simulink model "cable_robot_2t_4cables_2019b"  (R2019b)
settings: Solver=ode3  StartTime=0.0  StopTime=tend_sim  FixedStep=stepsize  MaxStep=1e-3  RelTol=1e-3
InitFcn:
  | close all
  | clear
  | Simulink.sdi.clear
  | run scripts\init_model.m
undefined symbols (not defined in the file): DirectionOfGravity, Dy0, f_max, f_min, g, K_fc, PlatformWeight, sigbuilder_block, T_fc, tend_sim, y0
settings Model: Creator=ac123748  LastModifiedBy=rausc
settings DataIOCC: SaveOutput=off  ReturnWorkspaceOutputs=off  SignalLoggingName=tmp_raccel_logsout
settings OptimizationCC: EfficientMapNaN2IntZero=off
settings DebuggingCC: ArithmeticOperatorsInVariantConditions=warning
settings HardwareCC: TargetBitPerPointer=64  TargetBitPerSizeT=64  TargetBitPerPtrDiffT=64  TargetLongLongMode=on  TargetIntDivRoundTo=Zero  TargetEndianess=LittleEndian  TargetWordSize=64  TargetHWDeviceType=MATLAB Host  ProdEqTarget=off
settings SFSimCC: SimUseLocalCustomCode=off  CustomCodeUndefinedFunction=UseInterfaceOnly
settings RTWCC: SystemTargetFile=raccel.tlc  TemplateMakefile=raccel_default_tmf  RTWVerbose=off  RTWUseLocalCustomCode=off  RTWUseSimCustomCode=on
settings CodeAppCC: GenerateComments=off  MaxIdLength=128  SimulinkBlockComments=off
settings RaccelTargetCC: LogVarNameModifier=rt_  MultiInstanceERTCode=off  ENABLE_SLEXEC_SSBRIDGE=0  RTWCAPISignals=off  RTWCAPIParams=off  RTWCAPIRootIO=off

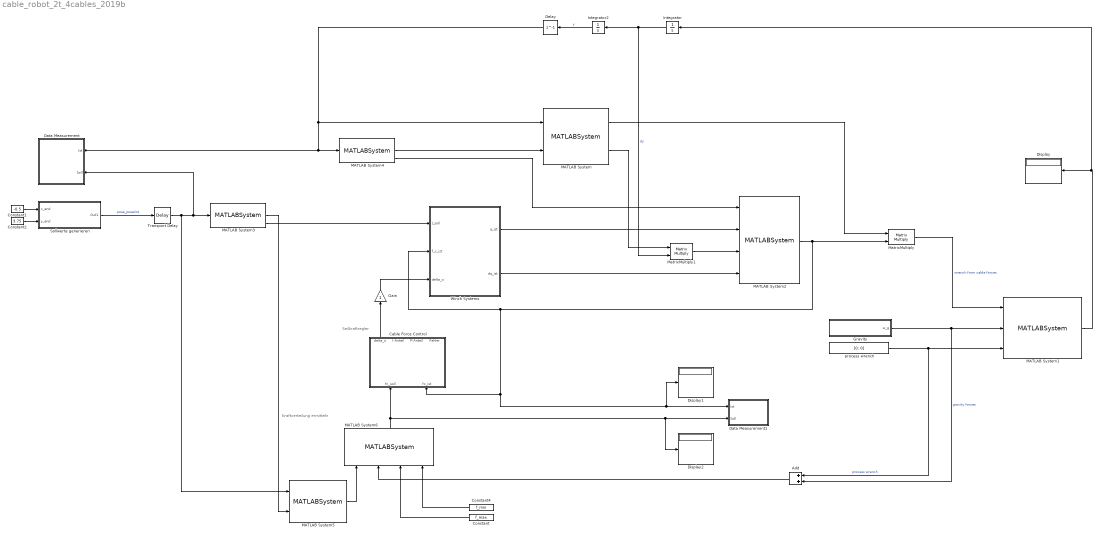
== system cable_robot_2t_4cables_2019b ==
  note: Seilkraftregler
  note: Kraftverteilung ermitteln
  Add : Sum
  Cable Force Control : Subsystem
  Constant : Constant  Value=f_max
  Constant1 : Constant  Value=-0.5
  Constant2 : Constant  Value=3.75
  Constant4 : Constant  Value=f_min
  Data Measurement : Subsystem
  Data Measurement1 : Subsystem
  Delay : Delay  DelayLength=1
  Display : Display
  Display1 : Display
  Display2 : Display
  Gain : Gain
  Gravity : Subsystem
  Integrator : Integrator  InitialCondition=Dy0
  Integrator2 : Integrator  InitialCondition=y0
  MATLAB System : MATLABSystem  System=sm.structurematrix_4cables  inv_Jacobian=on  Platform=zeros( 4, 2 )
      mask Type: sm.structurematrix_4cables
      mask Display:
      | disp('sm.structurematrix_4cables');
      | port_label('input',1,'p');
      | port_label('input',2,'u');
      | port_label('output',1,'AT');
      | port_label('output',2,'J_inv');
  MATLAB System1 : MATLABSystem  System=dynamics.platform_4cables  Weight=5
      mask Type: dynamics.platform_4cables
      mask Display:
      | disp('dynamics.platform_4cables');
      | port_label('input',1,'w_c');
      | port_label('input',2,'w_g');
      | port_label('input',3,'w_p');
      | port_label('output',1,'ddy');
  MATLAB System2 : MATLABSystem  System=cable.linearelasticity_4cables  Elasticity=172e3 * ones( 4, 1 )  Viscosity=0.03 * 172e3 * ones( 4, 1 )  Reference_Length=ones( 4, 1 )  Initial_Length=zeros( 4, 1 )  SimulateUsing=Code generation
      mask Type: cable.linearelasticity_4cables
      mask Display:
      | disp('cable.linearelasticity_4cables');
      | port_label('input',1,'l');
      | port_label('input',2,'q');
      | port_label('input',3,'dl');
      | port_label('input',4,'dq');
      | port_label('output',1,'f_c');
  MATLAB System3 : MATLABSystem  System=ik.ik_standard_4cables  UnitVectors=on  DeltaLength=on  FrameAnchors=[ [ -4.70, 4.30 ]; [ 3.70, 3.20 ]; [ 3.50, -5.20 ]; [ -4.50, -5.00 ] ]  Platform=zeros( 4, 2 )  InitialPose=zeros( 2, 1 )  CableOffset=zeros( 4, 1 )
      mask Type: ik.ik_standard_4cables
      mask Display:
      | disp('ik.ik_standard_4cables');
      | port_label('input',1,'p');
      | port_label('output',1,'l');
      | port_label('output',2,'u');
      | port_label('output',3,'delta_l');
  MATLAB System4 : MATLABSystem  System=ik.ik_standard_4cables  UnitVectors=on  DeltaLength=on  FrameAnchors=[ [ -4.70, 4.30 ]; [ 3.70, 3.20 ]; [ 3.50, -5.20 ]; [ -4.50, -5.00 ] ]  Platform=zeros( 4, 2 )  InitialPose=zeros( 2, 1 )  CableOffset=zeros( 4, 1 )
      mask Type: ik.ik_standard_4cables
      mask Display:
      | disp('ik.ik_standard_4cables');
      | port_label('input',1,'p');
      | port_label('output',1,'l');
      | port_label('output',2,'u');
      | port_label('output',3,'delta_l');
  MATLAB System5 : MATLABSystem  System=sm.structurematrix_4cables  inv_Jacobian=off  Platform=zeros( 4, 2 )
      mask Type: sm.structurematrix_4cables
      mask Display:
      | disp('sm.structurematrix_4cables');
      | port_label('input',1,'p');
      | port_label('input',2,'u');
      | port_label('output',1,'AT');
  MATLAB System6 : MATLABSystem  System=dynamics.call_closed_form
      mask Type: dynamics.call_closed_form
      mask Display:
      | disp('dynamics.call_closed_form');
      | port_label('input',1,'AT');
      | port_label('input',2,'w');
      | port_label('input',3,'f_max');
      | port_label('input',4,'f_min');
      | port_label('output',1,'f_c_soll');
  MatrixMultiply : Product  Multiplication=Matrix(*)
  MatrixMultiply1 : Product  Multiplication=Matrix(*)
  Sollwerte generieren : Subsystem
  Transport Delay : TransportDelay
  Winch Systems : Subsystem
  process wrench : Constant  Value=[0; 0]
  wires:
  Sollwerte generieren/1(Out1) -> Transport Delay/1  "pose_poselist"
  Transport Delay/1 -> MATLAB System5/1, MATLAB System3/1, Data Measurement/2(Soll)
  MATLAB System3/3 -> Winch Systems/1(l_soll)
  Winch Systems/2(dq_ist) -> MATLAB System2/4
  Winch Systems/1(q_ist) -> MATLAB System2/2
  MATLAB System/1 -> MatrixMultiply/1
  MATLAB System/2 -> MatrixMultiply1/1
  Gravity/1(w_g) -> Add/2, MATLAB System1/2  "gravity forces"
  process wrench/1 -> Add/1, MATLAB System1/3  "process wrench"
  MatrixMultiply/1 -> MATLAB System1/1  "wrench from cable forces"
  Integrator/1 -> MatrixMultiply1/2, Integrator2/1  "dy"
  Integrator2/1 -> Delay/1  "y"
  MATLAB System4/2 -> MATLAB System/2
  MATLAB System3/2 -> MATLAB System5/2
  Delay/1 -> MATLAB System4/1, Data Measurement/1(Ist), MATLAB System/1
  MATLAB System5/1 -> MATLAB System6/1
  MATLAB System6/1 -> Display2/1, Data Measurement1/2(Soll), Cable Force Control/1("fc_soll ")
  Constant4/1 -> MATLAB System6/4
  Constant/1 -> MATLAB System6/3
  Cable Force Control/1(delta_o) -> Gain/1
  Add/1 -> MATLAB System6/2
  MATLAB System2/1 -> Cable Force Control/2(fc_ist), Display1/1, Data Measurement1/1(Ist), Winch Systems/2(f_c_ist), MatrixMultiply/2
  Gain/1 -> Winch Systems/3(delta_o)
  MATLAB System1/1 -> Integrator/1, Display/1
  MATLAB System4/3 -> MATLAB System2/1
  MatrixMultiply1/1 -> MATLAB System2/3
  Constant1/1 -> Sollwerte generieren/1(x_end)
  Constant2/1 -> Sollwerte generieren/2(y_end)

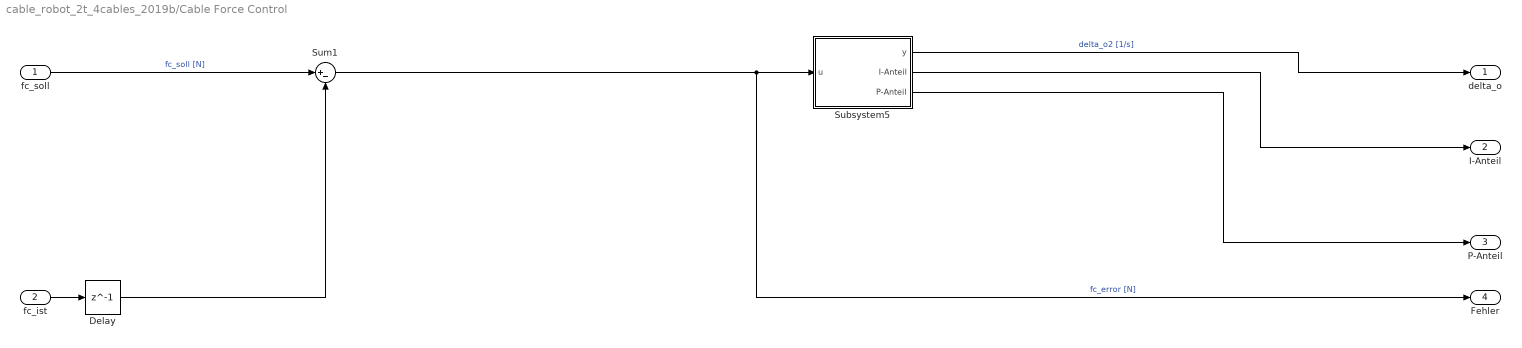
== system cable_robot_2t_4cables_2019b/Cable Force Control ==
  "fc_soll " : Inport
  fc_ist : Inport  Port=2
  Delay : Delay  DelayLength=1
  Subsystem5 : Subsystem  VariantControl=Choice
  Sum1 : Sum  Inputs=|+-
  delta_o : Outport
  I-Anteil : Outport  Port=2
  P-Anteil : Outport  Port=3
  Fehler : Outport  Port=4
  wires:
  Subsystem5/1(y) -> delta_o/1  "delta_o2 [1/s]"
  "fc_soll "/1 -> Sum1/1  "fc_soll [N]"
  Sum1/1 -> Fehler/1, Subsystem5/1(u)  "fc_error [N]"
  Subsystem5/2(I-Anteil) -> I-Anteil/1
  Subsystem5/3(P-Anteil) -> P-Anteil/1
  fc_ist/1 -> Delay/1
  Delay/1 -> Sum1/2

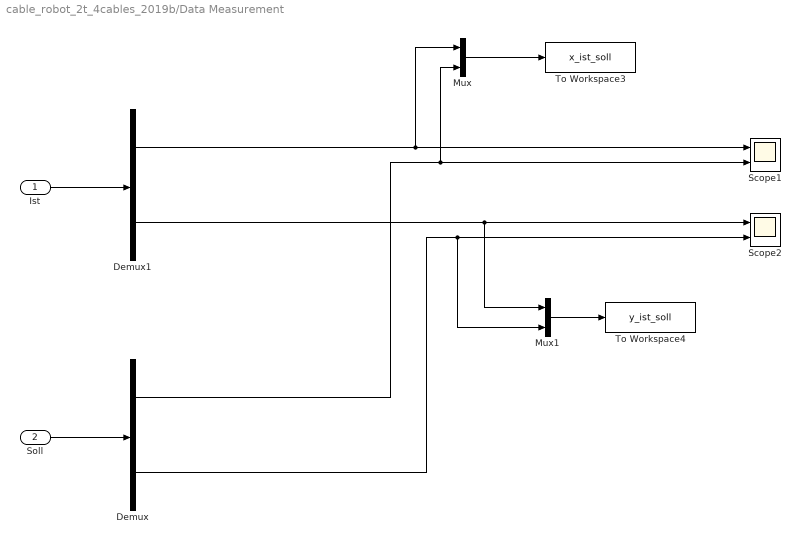
== system cable_robot_2t_4cables_2019b/Data Measurement ==
  Ist : Inport
  Soll : Inport  Port=2
  Demux : Demux  Outputs=2
  Demux1 : Demux  Outputs=2
  Mux : Mux  Inputs=2
  Mux1 : Mux  Inputs=2
  Scope1 : Scope  NumInputPorts=2
  Scope2 : Scope  NumInputPorts=2
  To Workspace3 : ToWorkspace  VariableName=x_ist_soll  SampleTime=-1
      settings: Decimation=1000  Save2DSignal=2-D array (concatenate along first dimension)
  To Workspace4 : ToWorkspace  VariableName=y_ist_soll  SampleTime=-1
      settings: Decimation=1000  Save2DSignal=2-D array (concatenate along first dimension)
  wires:
  Soll/1 -> Demux/1
  Ist/1 -> Demux1/1
  Demux1/1 -> Mux/1, Scope1/1
  Demux1/2 -> Mux1/1, Scope2/1
  Demux/2 -> Mux1/2, Scope2/2
  Demux/1 -> Mux/2, Scope1/2
  Mux/1 -> To Workspace3/1
  Mux1/1 -> To Workspace4/1

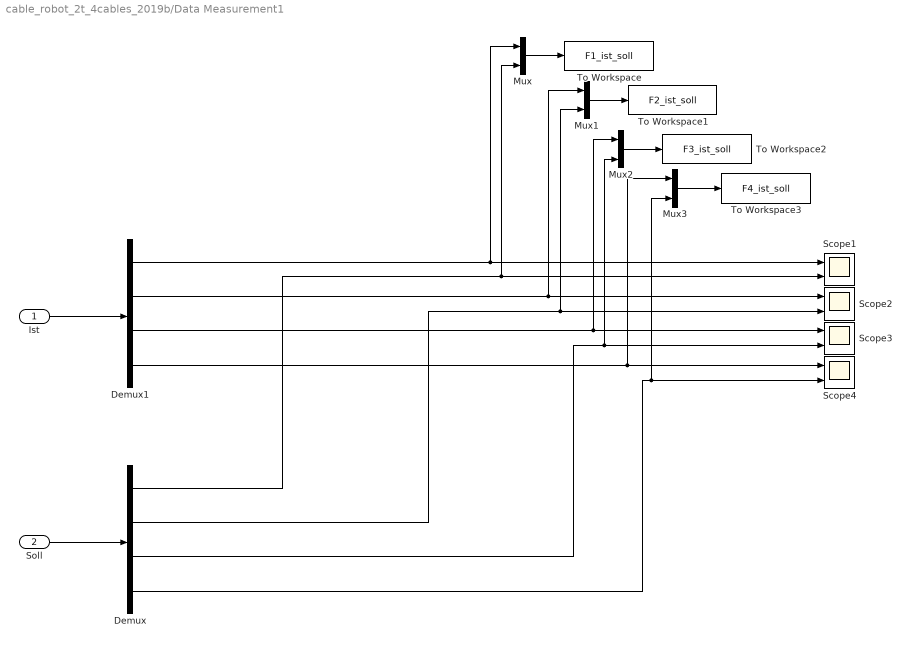
== system cable_robot_2t_4cables_2019b/Data Measurement1 ==
  Ist : Inport
  Soll : Inport  Port=2
  Demux : Demux
  Demux1 : Demux
  Mux{,1..3} (4 alike) : Mux  Inputs=2
  Scope{1..4} (4 alike) : Scope  NumInputPorts=2
  To Workspace : ToWorkspace  VariableName=F1_ist_soll  SampleTime=-1
      settings: Decimation=1000
  To Workspace1 : ToWorkspace  VariableName=F2_ist_soll  SampleTime=-1
      settings: Decimation=1000
  To Workspace2 : ToWorkspace  VariableName=F3_ist_soll  SampleTime=-1
      settings: Decimation=1000
  To Workspace3 : ToWorkspace  VariableName=F4_ist_soll  SampleTime=-1
      settings: Decimation=1000
  wires:
  Demux/1 -> Scope1/2, Mux/2
  Demux1/1 -> Scope1/1, Mux/1
  Ist/1 -> Demux1/1
  Soll/1 -> Demux/1
  Mux/1 -> To Workspace/1
  Mux1/1 -> To Workspace1/1
  Demux1/2 -> Scope2/1, Mux1/1
  Demux/2 -> Scope2/2, Mux1/2
  Demux/3 -> Mux2/2, Scope3/2
  Demux1/3 -> Mux2/1, Scope3/1
  Mux2/1 -> To Workspace2/1
  Mux3/1 -> To Workspace3/1
  Demux1/4 -> Mux3/1, Scope4/1
  Demux/4 -> Scope4/2, Mux3/2

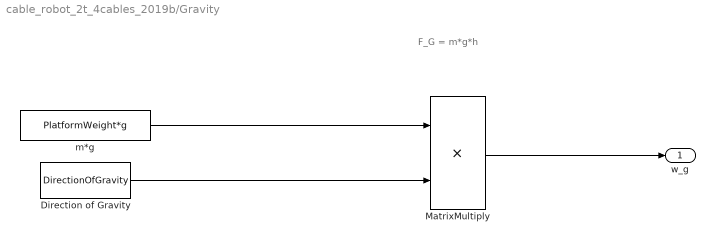
== system cable_robot_2t_4cables_2019b/Gravity ==
  note: F_G = m*g*h
  Direction of Gravity : Constant  Value=DirectionOfGravity
  MatrixMultiply : Product
  m*g : Constant  Value=PlatformWeight*g
  w_g : Outport
  wires:
  MatrixMultiply/1 -> w_g/1
  m*g/1 -> MatrixMultiply/1
  Direction of Gravity/1 -> MatrixMultiply/2

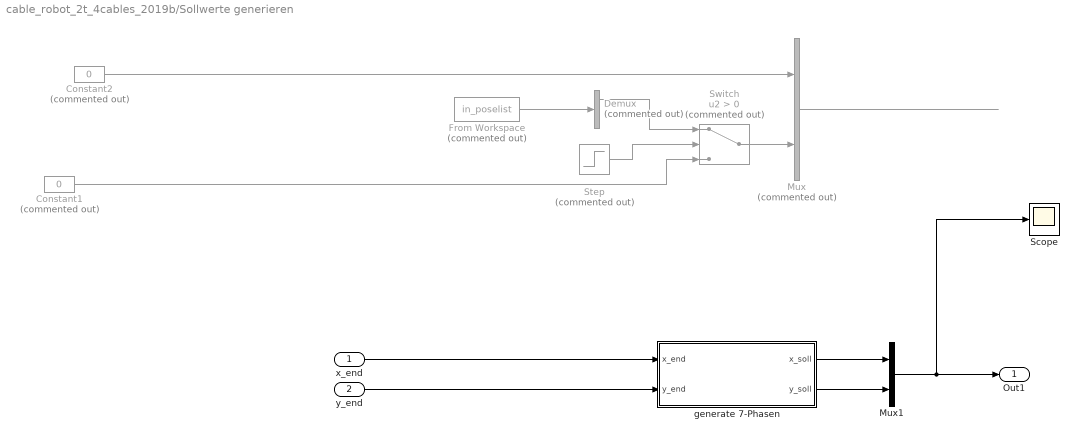
== system cable_robot_2t_4cables_2019b/Sollwerte generieren ==
  x_end : Inport
  y_end : Inport  Port=2
  Constant1 : Constant  Commented=on  Value=0
  Constant2 : Constant  Commented=on  Value=0
  Demux : Demux  Commented=on  Outputs=2
  From Workspace : FromWorkspace  Commented=on  VariableName=in_poselist
  Mux : Mux  Commented=on  Inputs=2
  Mux1 : Mux  Inputs=2
  Scope : Scope
  Step : Step  Commented=on  SampleTime=0
  Switch : Switch  Commented=on  Criteria=u2 > Threshold
  generate 7-Phasen : Subsystem
  Out1 : Outport
  wires:
  Mux/1 -> ?
  Constant2/1 -> Mux/1
  Constant1/1 -> Switch/3
  From Workspace/1 -> Demux/1
  Demux/1 -> Switch/1
  Switch/1 -> Mux/2
  Step/1 -> Switch/2
  generate 7-Phasen/1(x_soll) -> Mux1/1
  generate 7-Phasen/2(y_soll) -> Mux1/2
  Mux1/1 -> Scope/1, Out1/1
  x_end/1 -> generate 7-Phasen/1(x_end)
  y_end/1 -> generate 7-Phasen/2(y_end)

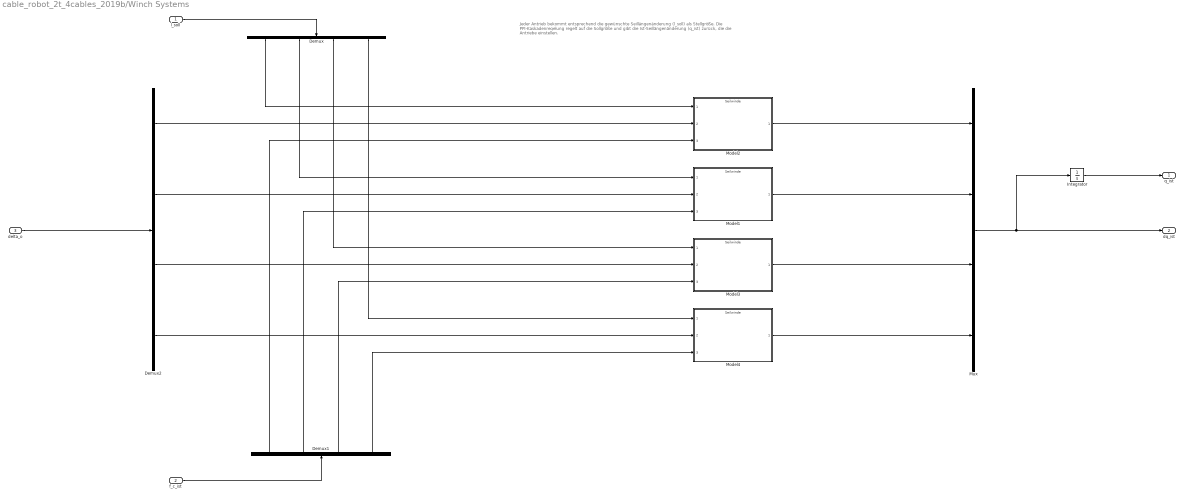
== system cable_robot_2t_4cables_2019b/Winch Systems ==
  note: Jeder Antrieb bekommt entsprechend die gewünschte Seillängenänderung (l_soll) als Stellgröße.
      | Die PPI-Kaskadenregelung regelt auf die Sollgröße und gibt die Ist-Seillängenänderung (q_ist) zurück,
      | die die Antriebe einstellen.
  l_soll : Inport
  f_c_ist : Inport  Port=2
  delta_o : Inport  Port=3
  Demux : Demux
  Demux1 : Demux
  Demux2 : Demux
  Integrator : Integrator
  Model{1..4} (4 alike) : ModelReference  ModelNameDialog=Seilwinde.slx  SimulationMode=Normal  ModelReferenceVersion=1.65
  Mux : Mux
  q_ist : Outport
  dq_ist : Outport  Port=2
  wires:
  Mux/1 -> Integrator/1, dq_ist/1
  Demux/1 -> Model2/1
  Model2/1 -> Mux/1
  Model1/1 -> Mux/2
  Model3/1 -> Mux/3
  Demux/3 -> Model3/1
  Demux/2 -> Model1/1
  Demux/4 -> Model4/1
  f_c_ist/1 -> Demux1/1
  Demux1/2 -> Model1/3
  Demux1/3 -> Model3/3
  Demux1/4 -> Model4/3
  l_soll/1 -> Demux/1
  Integrator/1 -> q_ist/1
  delta_o/1 -> Demux2/1
  Demux2/1 -> Model2/2
  Demux2/2 -> Model1/2
  Demux2/3 -> Model3/2
  Demux2/4 -> Model4/2
  Demux1/1 -> Model2/3
  Model4/1 -> Mux/4

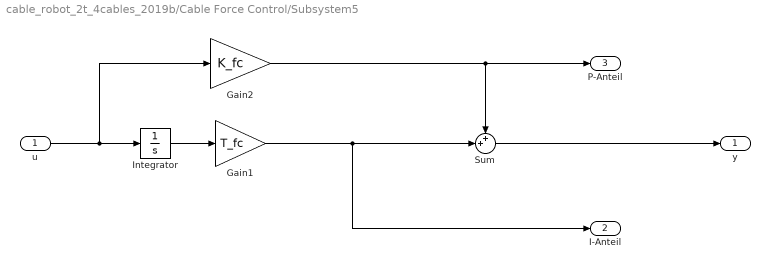
== system cable_robot_2t_4cables_2019b/Cable Force Control/Subsystem5 ==
  u : Inport
  Gain1 : Gain  Gain=T_fc
  Gain2 : Gain  Gain=K_fc
  Integrator : Integrator
  Sum : Sum  Inputs=++|
  y : Outport
  I-Anteil : Outport  Port=2
  P-Anteil : Outport  Port=3
  wires:
  Integrator/1 -> Gain1/1
  u/1 -> Gain2/1, Integrator/1
  Sum/1 -> y/1
  Gain1/1 -> Sum/2, I-Anteil/1
  Gain2/1 -> Sum/1, P-Anteil/1

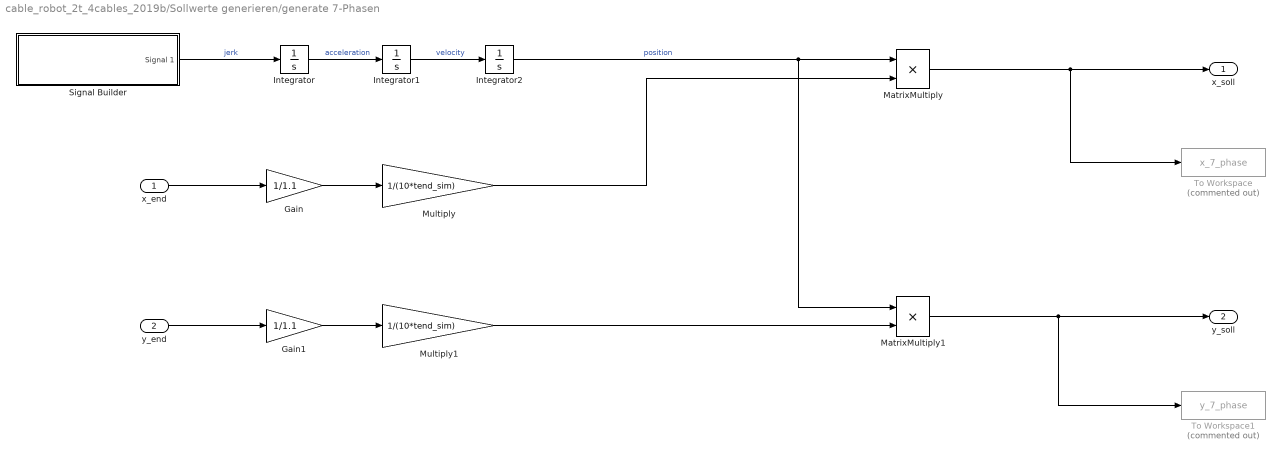
== system cable_robot_2t_4cables_2019b/Sollwerte generieren/generate 7-Phasen ==
  x_end : Inport
  y_end : Inport  Port=2
  Gain : Gain  Gain=1/1.1
  Gain1 : Gain  Gain=1/1.1
  Integrator : Integrator
  Integrator1 : Integrator
  Integrator2 : Integrator
  MatrixMultiply : Product
  MatrixMultiply1 : Product
  Multiply : Gain  Gain=1/(10*tend_sim)
  Multiply1 : Gain  Gain=1/(10*tend_sim)
  Signal Builder : Subsystem  Tag=STV Subsys  LoadFcn=sigbuilder_block('load');  StartFcn=sigbuilder_block('start');  StopFcn=sigbuilder_block('stop');  ClipboardFcn=sigbuilder_block('clipboard');  mask(Sigbuilder block){tuvar=[0:10]}
      mask help: Simulink:masks:SigbuilderBlock_MD
      mask init:
      | if ~strcmp(get_param(bdroot(gcbh),'SimulationStatus'),'stopped') tuvar = sigbuilder_block('maskInit'); end
      settings: CopyFcn=sigbuilder_block('copy');  DeleteFcn=sigbuilder_block('delete');  ModelCloseFcn=sigbuilder_block('modelClose');  PreSaveFcn=sigbuilder_block('preSave');  PauseFcn=sigbuilder_block('pause');  ContinueFcn=sigbuilder_block('continue');  NameChangeFcn=sigbuilder_block('namechange');  OpenFcn=sigbuilder_block('open',[6 30 1428 681.75 ]);  CloseFcn=sigbuilder_block('close');
      mask Display: plot(0, 0, 100, 100,[2, 2, 32, 32, 2], [68, 8, 8, 68, 68],[32, 2], [38, 38], [32, 19, 2],[53, 60, 44], [32, 17, 17, 2],[16, 16, 31, 31]);txt = getActiveGroup(gcbh);text(2, 100, txt,'verticalAlignment', 'top');
  To Workspace : ToWorkspace  Commented=on  VariableName=x_7_phase  SampleTime=-1
      settings: Save2DSignal=2-D array (concatenate along first dimension)
  To Workspace1 : ToWorkspace  Commented=on  VariableName=y_7_phase  SampleTime=-1
      settings: Save2DSignal=2-D array (concatenate along first dimension)
  x_soll : Outport
  y_soll : Outport  Port=2
  wires:
  Signal Builder/1(Signal 1) -> Integrator/1  "jerk"
  Integrator/1 -> Integrator1/1  "acceleration"
  Integrator1/1 -> Integrator2/1  "velocity"
  MatrixMultiply/1 -> To Workspace/1, x_soll/1
  MatrixMultiply1/1 -> y_soll/1, To Workspace1/1
  x_end/1 -> Gain/1
  Multiply/1 -> MatrixMultiply/2
  Integrator2/1 -> MatrixMultiply1/1, MatrixMultiply/1  "position"
  y_end/1 -> Gain1/1
  Multiply1/1 -> MatrixMultiply1/2
  Gain/1 -> Multiply/1
  Gain1/1 -> Multiply1/1

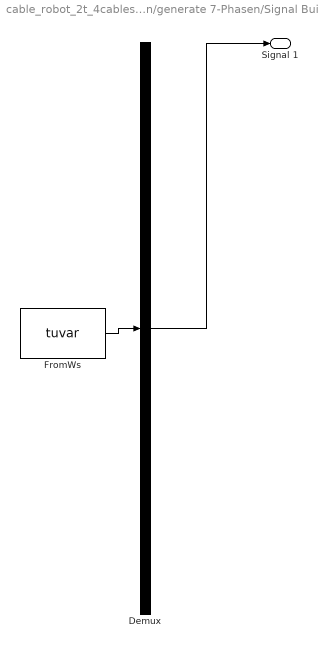
== system cable_robot_2t_4cables_2019b/Sollwerte generieren/generate 7-Phasen/Signal Builder ==
  Demux : Demux  Tag=STV Demux  Outputs=1
      settings: DisplayOption=none
  FromWs : FromWorkspace  Tag=STV FromWs  VariableName=tuvar
      SigBuilderData=|
      | common.afterFinalStr = 'Extrapolate'
      | common.sampleTime = 0
      | dataSet.timeRange = [0 20]
      | dataSet.name = 'Group 1'
      | sbobj.Groups.Name = 'Group 1'
      | sbobj.Groups.Signals.Name = 'Signal 1'
      | sbobj.Groups.Signals.XData = [0 3 3 6 6 9 9 12 12 15 15 18 18 20]
      | sbobj.Groups.Signals.YData = [1.01 1 0 0 -1 -1 0 0 -1 -1 0 0 1 1]
      | sbobj.Groups.TimeRange = [0 20]
  Signal 1 : Outport  Tag=STV Outport
  wires:
  Demux/1 -> Signal 1/1
  FromWs/1 -> Demux/1
